simulink model "quarter_sus_imp_force"  (R2025a)
settings: Solver=FixedStepAuto  StartTime=0.0  StopTime=20  FixedStep=0.001  RelTol=1e-3
model workspace (MAT data in the model file):
  Cs : Simulink.Parameter (value not decoded)
  Cy_f1 = 128915.5
  Cy_r1 = 85943.6
  G0 : Simulink.Parameter (value not decoded)
  IDA_ISD_PBC_bd : Simulink.Parameter (value not decoded)
  IDA_ISD_PBC_c1 : Simulink.Parameter (value not decoded)
  IDA_ISD_PBC_k1 : Simulink.Parameter (value not decoded)
  IDA_ISD_PBC_k2 : Simulink.Parameter (value not decoded)
  IDA_ISD_PBC_r1 : Simulink.Parameter (value not decoded)
  IDA_PBC_cd4 = 2000
  IDA_PBC_kd2 = 10000
  IDA_PBC_r1 = 1.5
  IDA_PBC_r2 = 0.44
  ISD_1_b : Simulink.Parameter (value not decoded)
  ISD_1_c : Simulink.Parameter (value not decoded)
  ISD_1_k1 : Simulink.Parameter (value not decoded)
  ISD_1_k2 : Simulink.Parameter (value not decoded)
  Izz1 = 1536.7
  Ks : Simulink.Parameter (value not decoded)
  Kt : Simulink.Parameter (value not decoded)
  Q : Simulink.Parameter (value not decoded)
  Q_F : Simulink.Parameter (value not decoded)
  Q_b_deflec : Simulink.Parameter (value not decoded)
  Q_delta_F : Simulink.Parameter (value not decoded)
  Q_dot : Simulink.Parameter (value not decoded)
  Q_dot_s : Simulink.Parameter (value not decoded)
  Q_dot_s_h : Simulink.Parameter (value not decoded)
  Q_dot_u : Simulink.Parameter (value not decoded)
  Q_flec : Simulink.Parameter (value not decoded)
  Q_flec_t : Simulink.Parameter (value not decoded)
  SHADD_alpha : Simulink.Parameter (value not decoded)
  a1 = 1.015
  a_max : Simulink.Parameter (value not decoded)
  a_min : Simulink.Parameter (value not decoded)
  adva_max : Simulink.Parameter (value not decoded)
  adva_min : Simulink.Parameter (value not decoded)
  as_max : Simulink.Parameter (value not decoded)
  b1 = 1.895
  b_deflec : Simulink.Parameter (value not decoded)
  bump_height : Simulink.Parameter (value not decoded)
  bump_lenth : Simulink.Parameter (value not decoded)
  bump_start : Simulink.Parameter (value not decoded)
  damper_param : Simulink.Parameter (value not decoded)
  deflec_max : Simulink.Parameter (value not decoded)
  done_range : Simulink.Parameter (value not decoded)
  f0 : Simulink.Parameter (value not decoded)
  h1 = 0.54
  imp_Cs : Simulink.Parameter (value not decoded)
  imp_Ks : Simulink.Parameter (value not decoded)
  imp_Ms : Simulink.Parameter (value not decoded)
  inerter_b : Simulink.Parameter (value not decoded)
  inerter_b_2 : Simulink.Parameter (value not decoded)
  inerter_c : Simulink.Parameter (value not decoded)
  inerter_k : Simulink.Parameter (value not decoded)
  inerter_k_2 : Simulink.Parameter (value not decoded)
  ms : Simulink.Parameter (value not decoded)
  mu : Simulink.Parameter (value not decoded)
  noise_seed : Simulink.Parameter (value not decoded)
  omega_1 : Simulink.Parameter (value not decoded)
  omega_2 : Simulink.Parameter (value not decoded)
  omega_3 : Simulink.Parameter (value not decoded)
  omega_4 : Simulink.Parameter (value not decoded)
  omega_5 : Simulink.Parameter (value not decoded)
  punish_Q : Simulink.Parameter (value not decoded)
  punish_R : Simulink.Parameter (value not decoded)
  reward_w_as : Simulink.Parameter (value not decoded)
  reward_w_au : Simulink.Parameter (value not decoded)
  reward_w_defv : Simulink.Parameter (value not decoded)
  road_seed : Simulink.Parameter (value not decoded)
  road_type : Simulink.Parameter (value not decoded)
  sigma_f1 = 0.1
  sigma_r1 = 0.1
  sine_amp : Simulink.Parameter (value not decoded)
  sine_freq : Simulink.Parameter (value not decoded)
  u : Simulink.Parameter (value not decoded)
  vs0 : Simulink.Parameter (value not decoded)
  vu0 : Simulink.Parameter (value not decoded)
  x_max : Simulink.Parameter (value not decoded)
  x_min : Simulink.Parameter (value not decoded)
  xs0 : Simulink.Parameter (value not decoded)
  xu0 : Simulink.Parameter (value not decoded)
symbols that are objects in the model workspace (value not decoded): a_max, a_min, b_deflec, bump_height, bump_lenth, bump_start, Cs, damper_param, f0, G0, IDA_ISD_PBC_bd, IDA_ISD_PBC_c1, IDA_ISD_PBC_k1, IDA_ISD_PBC_k2, IDA_ISD_PBC_r1, imp_Cs, imp_Ks, imp_Ms, Ks, Kt, ms, mu, omega_1, omega_2, omega_3, omega_4, omega_5, Q_b_deflec, Q_delta_F, Q_dot_s, Q_dot_s_h, Q_dot_u, Q_F, Q_flec, Q_flec_t, road_type, SHADD_alpha, sine_amp, sine_freq, vs0, vu0, xs0, xu0
undefined symbols (not defined in the file): ADD, Force, IDA, Imp, Imp_Force, PBC, SH, Train, Validation
libraries: fl_lib x32, nesl_utility x27, sharedTrackingLibrary x4, sdl_lib x2, dspstat3 x2, deeplib x1, simulink x1
(part 2 of 6)

== system quarter_sus_imp_force/QuarterSuspension /reward_cal/reward_cal ==
  state : Inport
  info : Inport  Port=2
  Add : Sum
  Add1 : Sum  Inputs=+-
  Add2 : Sum
  Constant1 : Constant  Value=Q_flec
  Constant3 : Constant  Value=b_deflec
  Demux : Demux  Outputs=2
  Gain : Gain  Gain=Q_dot_s
  Gain1 : Gain  Gain=Q_dot_u
  Gain2 : Gain  Gain=-1
  Selector : Selector  InputPortWidth=8  IndexOptions=Index vector (dialog)  Indices=[7 8]  OutputSizes=1
  Selector1 : Selector  InputPortWidth=4  IndexOptions=Index vector (dialog)  Indices=[1]  OutputSizes=1
  Selector2 : Selector  InputPortWidth=4  IndexOptions=Index vector (dialog)  Indices=[3]  OutputSizes=1
  Square : Math  Operator=square
  Square1 : Math  Operator=square
  cal_reward : MATLAB Function  TreatAsAtomicUnit=on
  reward : Outport
  wires:
  Constant1/1 -> cal_reward/3(Q_flec)
  Constant3/1 -> cal_reward/2(b_def)
  cal_reward/1(reward) -> Add/1  "reward_deflec"
  Add/1 -> Gain2/1  "reward"
  Add2/1 -> Add/2  "reward_dot"
  state/1 -> Selector2/1, Selector1/1
  Selector2/1 -> Add1/2
  Selector1/1 -> Add1/1
  Add1/1 -> cal_reward/1(state_deflec)
  info/1 -> Selector/1
  Selector/1 -> Demux/1
  Demux/1 -> Square/1
  Demux/2 -> Square1/1
  Square/1 -> Gain/1
  Square1/1 -> Gain1/1
  Gain2/1 -> reward/1
  Gain/1 -> Add2/1  "reward_accs"
  Gain1/1 -> Add2/2  "reward_accu"

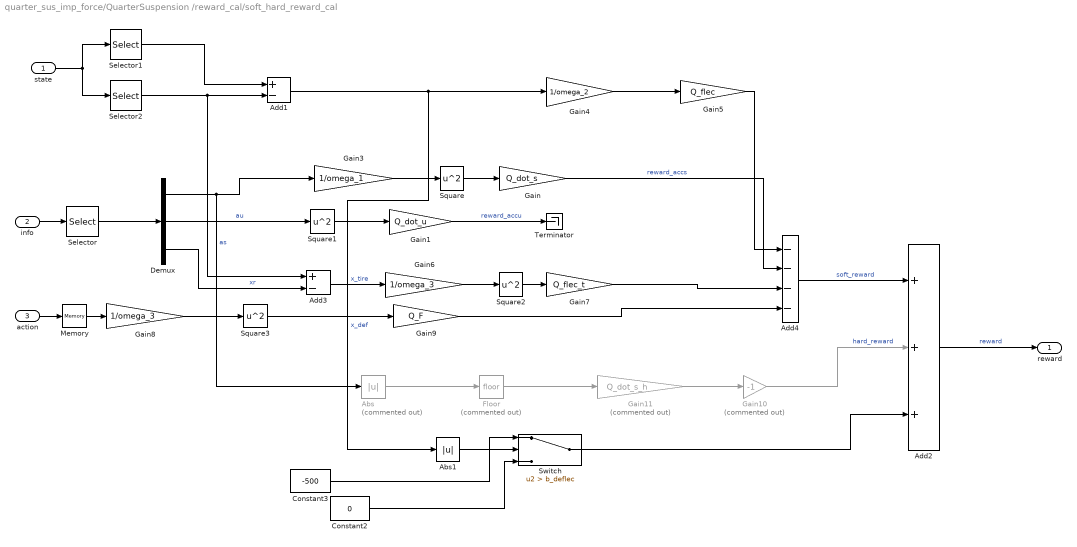
== system quarter_sus_imp_force/QuarterSuspension /reward_cal/soft_hard_reward_cal ==
  state : Inport
  info : Inport  Port=2
  action : Inport  Port=3
  Abs : Abs  Commented=on  SaturateOnIntegerOverflow=off
  Abs1 : Abs  SaturateOnIntegerOverflow=off
  Add1 : Sum  Inputs=+-
  Add2 : Sum  Inputs=+++
  Add3 : Sum  Inputs=+-
  Add4 : Sum  Inputs=----
  Constant2 : Constant  Value=0
  Constant3 : Constant  Value=-500
  Demux : Demux  Outputs=3
  Floor : Rounding  Commented=on
  Gain : Gain  Gain=Q_dot_s
  Gain1 : Gain  Gain=Q_dot_u
  Gain10 : Gain  Commented=on  Gain=-1
  Gain11 : Gain  Commented=on  Gain=Q_dot_s_h
  Gain3 : Gain  Gain=1/omega_1
  Gain4 : Gain  Gain=1/omega_2
  Gain5 : Gain  Gain=Q_flec
  Gain6 : Gain  Gain=1/omega_3
  Gain7 : Gain  Gain=Q_flec_t
  Gain8 : Gain  Gain=1/omega_3
  Gain9 : Gain  Gain=Q_F
  Memory : Memory
  Selector : Selector  InputPortWidth=8  IndexOptions=Index vector (dialog)  Indices=[7 8 6]  OutputSizes=1
  Selector1 : Selector  InputPortWidth=4  IndexOptions=Index vector (dialog)  Indices=[1]  OutputSizes=1
  Selector2 : Selector  InputPortWidth=4  IndexOptions=Index vector (dialog)  Indices=[3]  OutputSizes=1
  Square{,1..3} (4 alike) : Math  Operator=square
  Switch : Switch  Criteria=u2 > Threshold  Threshold=b_deflec  SaturateOnIntegerOverflow=off  InputSameDT=off
  Terminator : Terminator
  reward : Outport
  wires:
  Gain1/1 -> Terminator/1  "reward_accu"
  Gain/1 -> Add4/2  "reward_accs"
  Square1/1 -> Gain1/1
  Square/1 -> Gain/1
  Demux/2 -> Square1/1  "au"
  Demux/1 -> Abs/1, Gain3/1  "as"
  Selector/1 -> Demux/1
  info/1 -> Selector/1
  Add1/1 -> Abs1/1, Gain4/1  "x_def"
  Selector1/1 -> Add1/1
  Selector2/1 -> Add3/1, Add1/2
  state/1 -> Selector2/1, Selector1/1
  Add2/1 -> reward/1  "reward"
  Constant3/1 -> Switch/1
  Demux/3 -> Add3/2  "xr"
  Add3/1 -> Gain6/1  "x_tire"
  Gain3/1 -> Square/1
  Gain4/1 -> Gain5/1
  Gain6/1 -> Square2/1
  Square2/1 -> Gain7/1
  Gain7/1 -> Add4/3
  action/1 -> Memory/1
  Gain8/1 -> Square3/1
  Square3/1 -> Gain9/1
  Gain9/1 -> Add4/4
  Add4/1 -> Add2/1  "soft_reward"
  Abs/1 -> Floor/1
  Floor/1 -> Gain11/1
  Gain10/1 -> Add2/2  "hard_reward"
  Gain11/1 -> Gain10/1
  Switch/1 -> Add2/3
  Abs1/1 -> Switch/2
  Constant2/1 -> Switch/3
  Gain5/1 -> Add4/1
  Memory/1 -> Gain8/1

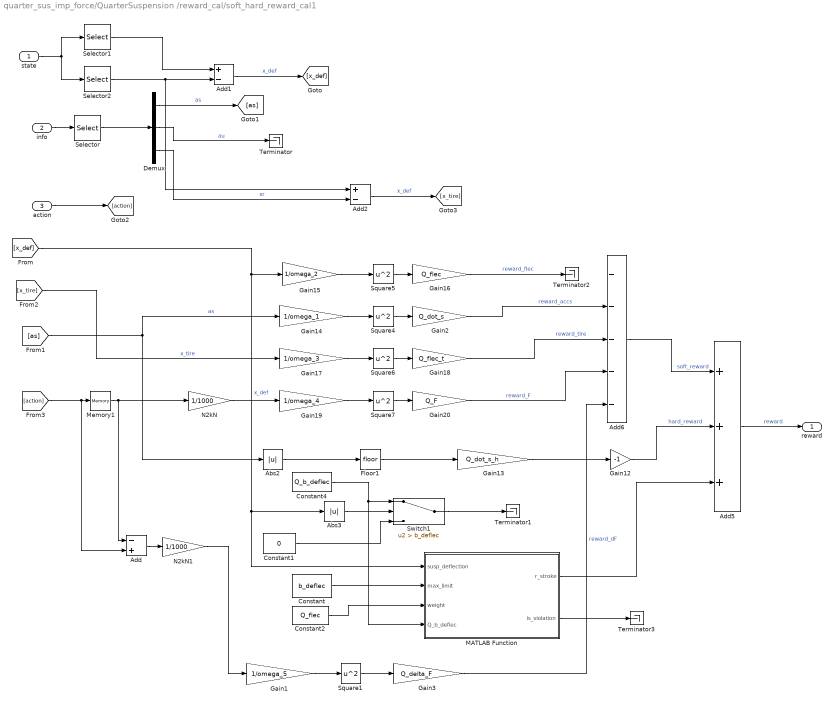
== system quarter_sus_imp_force/QuarterSuspension /reward_cal/soft_hard_reward_cal1 ==
  state : Inport
  info : Inport  Port=2
  action : Inport  Port=3
  Abs2 : Abs  SaturateOnIntegerOverflow=off
  Abs3 : Abs  SaturateOnIntegerOverflow=off
  Add : Sum  Inputs=-+
  Add1 : Sum  Inputs=+-
  Add2 : Sum  Inputs=+-
  Add5 : Sum  Inputs=+++
  Add6 : Sum  Inputs=-----
  Constant : Constant  Value=b_deflec
  Constant1 : Constant  Value=0
  Constant2 : Constant  Value=Q_flec
  Constant4 : Constant  Value=Q_b_deflec
  Demux : Demux  Outputs=3
  Floor1 : Rounding
  Gain1 : Gain  Gain=1/omega_5
  Gain12 : Gain  Gain=-1
  Gain13 : Gain  Gain=Q_dot_s_h
  Gain14 : Gain  Gain=1/omega_1
  Gain15 : Gain  Gain=1/omega_2
  Gain16 : Gain  Gain=Q_flec
  Gain17 : Gain  Gain=1/omega_3
  Gain18 : Gain  Gain=Q_flec_t
  Gain19 : Gain  Gain=1/omega_4
  Gain2 : Gain  Gain=Q_dot_s
  Gain20 : Gain  Gain=Q_F
  Gain3 : Gain  Gain=Q_delta_F
  MATLAB Function : MATLAB Function  TreatAsAtomicUnit=on
  Memory1 : Memory
  N2kN : Gain  Gain=1/1000
  N2kN1 : Gain  Gain=1/1000
  Selector : Selector  InputPortWidth=8  IndexOptions=Index vector (dialog)  Indices=[7 8 6]  OutputSizes=1
  Selector1 : Selector  InputPortWidth=4  IndexOptions=Index vector (dialog)  Indices=[1]  OutputSizes=1
  Selector2 : Selector  InputPortWidth=4  IndexOptions=Index vector (dialog)  Indices=[3]  OutputSizes=1
  Square{1,4..7} (5 alike) : Math  Operator=square
  Switch1 : Switch  Criteria=u2 > Threshold  Threshold=b_deflec  SaturateOnIntegerOverflow=off  InputSameDT=off
  Terminator{,1..3} (4 alike) : Terminator
  reward : Outport
  wires:
  action/1 -> [action]
  state/1 -> Selector1/1, Selector2/1
  Selector2/1 -> Add2/1, Add1/2
  Selector1/1 -> Add1/1
  Add1/1 -> [x_def]  "x_def"
  info/1 -> Selector/1
  Selector/1 -> Demux/1
  Demux/1 -> [as]  "as"
  Gain13/1 -> Gain12/1
  Gain19/1 -> Square7/1
  [x_tire] -> Gain17/1  "x_tire"
  Gain2/1 -> Add6/2  "reward_accs"
  Gain18/1 -> Add6/3  "reward_tire"
  Memory1/1 -> N2kN/1, Add/1
  Gain12/1 -> Add5/2  "hard_reward"
  Add6/1 -> Add5/1  "soft_reward"
  Constant1/1 -> Switch1/3
  Square4/1 -> Gain2/1
  Floor1/1 -> Gain13/1
  Gain20/1 -> Add6/4  "reward_F"
  Gain16/1 -> Terminator2/1  "reward_flec"
  [x_def] -> Gain15/1, MATLAB Function/1(susp_deflection), Abs3/1  "x_def"
  Gain17/1 -> Square6/1
  Abs2/1 -> Floor1/1
  Square7/1 -> Gain20/1
  [action] -> Add/2, Memory1/1
  Switch1/1 -> Terminator1/1
  Abs3/1 -> Switch1/2
  [as] -> Gain14/1, Abs2/1  "as"
  Add5/1 -> reward/1  "reward"
  Square5/1 -> Gain16/1
  Gain15/1 -> Square5/1
  Constant4/1 -> MATLAB Function/4(Q_b_deflec), Switch1/1
  Square6/1 -> Gain18/1
  N2kN/1 -> Gain19/1
  Gain14/1 -> Square4/1
  Demux/3 -> Add2/2  "xr"
  Add2/1 -> [x_tire]  "x_def"
  Demux/2 -> Terminator/1  "au"
  MATLAB Function/1(r_stroke) -> Add5/3
  Constant/1 -> MATLAB Function/2(max_limit)
  Constant2/1 -> MATLAB Function/3(weight)
  MATLAB Function/2(is_violation) -> Terminator3/1
  Add/1 -> N2kN1/1
  N2kN1/1 -> Gain1/1
  Gain1/1 -> Square1/1
  Square1/1 -> Gain3/1
  Gain3/1 -> Add6/5  "reward_dF"
